simulink model "SVPWM_code"  (Simulink 9.0)
settings: Solver=VariableStepAuto  StartTime=0.0  StopTime=10.0  RelTol=1e-3
settings Model: Creator=80573  LastModifiedBy=80573
settings DataIOCC: SaveFormat=Dataset
settings OptimizationCC: LifeSpan=auto
settings DebuggingCC: UnderspecifiedInitializationDetection=Simplified  MergeDetectMultiDrivingBlocksExec=error  SFUnexpectedBacktrackingDiag=error  SFNoUnconditionalDefaultTransitionDiag=error  SFExecutionAtInitializationDiag=warning
settings HardwareCC: ProdBitPerPointer=64  ProdBitPerSizeT=64  ProdBitPerPtrDiffT=64  ProdLargestAtomicFloat=Float  ProdIntDivRoundTo=Zero  ProdEndianess=LittleEndian  ProdWordSize=64  ProdHWDeviceType=Intel->x86-64 (Windows64)
settings ModelReferenceCC: PropagateSignalLabelsOutOfModel=on
settings CodeAppCC: StateflowObjectComments=off
settings GRTTargetCC: TargetLangStandard=C99 (ISO)
settings ConfigComp: CovMetricSettings=dwe  CovHtmlReporting=off  CovSaveCumulativeToWorkspaceVar=off  CovSaveSingleToWorkspaceVar=off  CovExternalEMLEnable=on

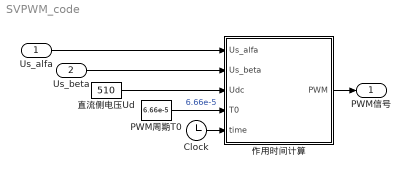
== system SVPWM_code ==
  Us_alfa : Inport
  Us_beta : Inport  Port=2
  Clock : Clock
  PWM周期T0 : Constant  Value=6.66e-5
  作用时间计算 : MATLAB Function  TreatAsAtomicUnit=on
  直流侧电压Ud : Constant  Value=510
  PWM信号 : Outport
  wires:
  Us_alfa/1 -> 作用时间计算/1(Us_alfa)
  作用时间计算/1(PWM) -> PWM信号/1
  Us_beta/1 -> 作用时间计算/2(Us_beta)
  直流侧电压Ud/1 -> 作用时间计算/3(Udc)
  PWM周期T0/1 -> 作用时间计算/4(T0)  "6.66e-5"
  Clock/1 -> 作用时间计算/5(time)

== matlab function 作用时间计算 ==
  data: Us_alfa input double; PWM output double; Us_beta input double; Udc input double; T0 input double; time input double
function PWM  = fcn(Us_alfa,Us_beta,Udc,T0,time)
% This block supports an embeddable subset of the MATLAB language.
% See the help menu for details.
%--------------------为了方便推导作用时间做出的设定值------------------------
X=sqrt(3)*T0*Us_beta/Udc;                           
Y=sqrt(3)/2*T0*Us_beta/Udc+3/2*T0*Us_alfa/Udc;     
Z=sqrt(3)/2*T0*Us_beta/Udc-3/2*T0*Us_alfa/Udc;      
%--------------------------------扇区值判断---------------------------------
%Uref1*sqrt(3)
%(Uref1+Uref2)*sqrt(3)
%(Uref1+Uref3)*sqrt(3)
%--------------------------------------------------------------------------
if(Us_beta>0)                                       %Uref1>0
    A=1;
else
    A=0;
end                                                                                                                                                                                                                                                                                                                                                                                                                                                                                                                                                                                                                                                                                                                                                                                                                                                                                                                                                                                                                                                                                                                                                                                                                                                                                   
if((sqrt(3)*Us_alfa-Us_beta)>0)                     %Uref2>0
    B=1;
else
    B=0; 
end
if((-sqrt(3)*Us_alfa-Us_beta)>0)                    %%Uref3>0
    C=1;
else
    C=0;
end
N=A+2*B+4*C;                                        %扇区值N，而不是扇区编号！！！！！！！
%--------------------------------------------------------------------------
%-----------------------------------分割线----------------------------------

%-----------------------------矢量作用时间计算-------------------------------
%--------------------------------S为扇区编号-------------------------------
switch(N)
    case 1
        S=2;%----------------------扇区编号S---------------------------
        t1=Z; 
        t2=Y; 
    case 2
        S=6;
        t1=Y; 
        t2=-X;
    case 3
        S=1;
        t1=-Z; 
        t2=X;
    case 4
        S=4;
        t1=-X; 
        t2=Z;
    case 5
        S=3;
        t1=X; 
        t2=-Y;
    case 6
        S=5;
        t1=-Y; 
        t2=-Z;
    otherwise
        S=1;
        t1=0; 
        t2=0;        
end
%--------------------------------------------------------------------------
%-----------------------------是否需要调制判断------------------------------
if((t1+t2)>T0)
    t11=t1*T0/(t1+t2);
    t21=t2*T0/(t1+t2);
    t1=t11;
    t2=t21;
    t0=0;
else
t0=T0-t1-t2;
end
%------------------------------------------------------------------------------------------------------------------------
%------------------------------普通定义电压---------------------------------
%U0=[0 0 0];U1=[1 0 0];U2=[1 1 0];U3=[0 1 0];
%U4=[0 1 1];U5=[0 0 1];U6=[1 0 1];U7=[1 1 1];
%------------------------由上可得八种电压输出信号控制（每种后面取反）---------
U0=[0 1 0 1 0 1];U1=[1 0 0 1 0 1];U2=[1 0 1 0 0 1];U3=[0 1 1 0 0 1];
U4=[0 1 1 0 1 0];U5=[0 1 0 1 1 0];U6=[1 0 0 1 1 0];U7=[1 0 1 0 1 0];
%--------------------------------------------------------------------------
t0=T0-t1-t2;
Ta=t0/4;
Tb=Ta+t1/2;
Tc=Tb+t2/2;
t=rem(time,T0);%t=时间time/周期Ts的余数 即在每个周期内作用的时间轴时间t
G=U0;
%------------------------------扇区编号S------------------------------------
%-------------------------------分割线--------------------------------------
switch (S)
    case 1
        G1=U1;
        G2=U2;
    case 2
        G1=U3;
        G2=U2;
    case 3
        G1=U3;
        G2=U4;
    case 4
        G1=U5;
        G2=U4;
    case 5
        G1=U5;
        G2=U6;
    case 6
        G1=U1;
        G2=U6;
    otherwise
        G1=U0;
        G2=U7;
end
%---------------------------七步分量法--------------------------------------
if (t<Ta)
	G=U0;       
elseif((t>=Ta)&&(t<Tb))
    G=G1;
elseif((t>=Tb)&&(t<Tc))
    G=G2;
elseif((t>=Tc)&&(t<(T0-Tc)))
    G=U7;
elseif((t>=(T0-Tc))&&(t<(T0-Tb)))
    G=G2;
elseif((t>=(T0-Tb))&&(t<(T0-Ta)))
    G=G1;
elseif((t>=(T0-Ta))&&(t<T0))
    G=U0;
end
PWM=G;
end
